simulink model "quizq2a"  (R2013b)
settings: Solver=ode4  StartTime=0.0  StopTime=25  RelTol=1e-3
values from neighbouring files (symbols this model uses):
  A = [0 1 0 0 0 0 ... (first row only)    [quizq2a.m]
  B = [0;1/m1;0;0;0;0]    [quizq2a.m]
  C = [0 1 0 0 0 0 ... (first row only)    [quizq2a.m]
  D = [0;0]    [quizq2a.m]
settings Model: Creator=makha  LastModifiedBy=Zeerak Nadeem Wyne
settings DataIOCC: LimitDataPoints=off  SaveFormat=Dataset
settings OptimizationCC: LifeSpan=auto  SimCompilerOptimization=off
settings DebuggingCC: UnderspecifiedInitializationDetection=Simplified  MergeDetectMultiDrivingBlocksExec=error  SolverPrmCheckMsg=none  FcnCallInpInsideContextMsg=error  FrameProcessingCompatibilityMsg=error  LibraryContextMissingDiagnostic=warning  SFUnexpectedBacktrackingDiag=error  SFNoUnconditionalDefaultTransitionDiag=error
settings HardwareCC: ProdBitPerPointer=64  ProdLargestAtomicFloat=Float  ProdIntDivRoundTo=Zero  ProdEndianess=LittleEndian  ProdWordSize=64  ProdHWDeviceType=Intel->x86-64 (Windows64)
settings ModelReferenceCC: PropagateSignalLabelsOutOfModel=on
settings SFSimCC: SimUseLocalCustomCode=on
settings RTWCC: RTWUseLocalCustomCode=on  RTWCompilerOptimization=off
settings GRTTargetCC: CodeReplacementLibrary=None  GeneratePreprocessorConditionals=Use local settings  CPPClassGenCompliant=on

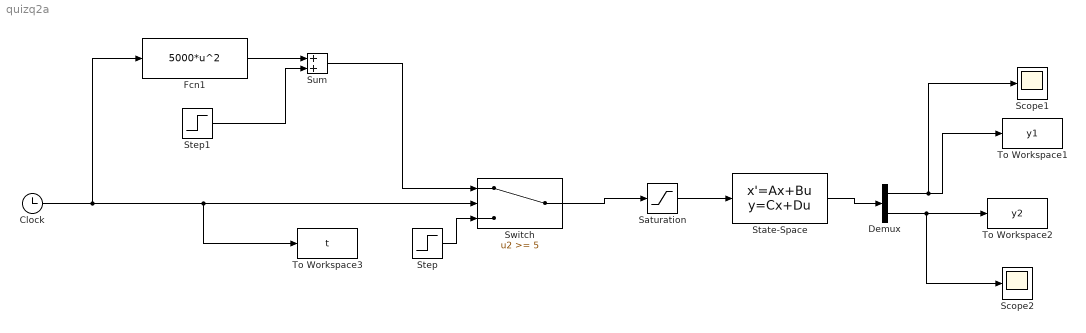
== system quizq2a ==
  Clock : Clock
      settings: Decimation=1000
  Demux : Demux  Outputs=2
  Fcn1 : Fcn  Expr=5000*u^2
  Saturation : Saturate  UpperLimit=2.2*10^6
  Scope1 : Scope
  Scope2 : Scope
      settings: SaveName=ScopeData2
  State-Space : StateSpace  A=A  B=B  C=C  D=D
  Step : Step  Time=0  After=3.25*10^3  SampleTime=0
  Step1 : Step  Time=5  After=2*10^5  SampleTime=0
  Sum : Sum
  Switch : Switch  Threshold=5  SaturateOnIntegerOverflow=off  InputSameDT=off
  To Workspace1 : ToWorkspace  VariableName=y1  SampleTime=-1
  To Workspace2 : ToWorkspace  VariableName=y2  SampleTime=-1
  To Workspace3 : ToWorkspace  VariableName=t  SampleTime=-1
  wires:
  Demux/1 -> Scope1/1, To Workspace1/1
  Demux/2 -> Scope2/1, To Workspace2/1
  State-Space/1 -> Demux/1
  Saturation/1 -> State-Space/1
  Switch/1 -> Saturation/1
  Sum/1 -> Switch/1
  Step1/1 -> Sum/2
  Fcn1/1 -> Sum/1
  Step/1 -> Switch/3
  Clock/1 -> Fcn1/1, To Workspace3/1, Switch/2
